simulink model "simulation_Hippocampus_compare_paper"  (R2022b)
settings: Solver=ode3  StartTime=0  StopTime=120  FixedStep=0.001  MaxStep=0.001  MinStep=0.00001  RelTol=1e-5  AbsTol=1e-5  EnableMultiTasking=on
values from neighbouring files (symbols this model uses):
  k_pos_ndi = 8    [parameters.m]
  k_vel_ndi = 8    [parameters.m]
  Kf = 6    [parameters.m]
  Kp = 0.01    [parameters.m]
  Kp_p = 30    [parameters.m]
  Kp_pitch = 8    [parameters.m]
  Kp_q = 10    [parameters.m]
  Kp_r = 10    [parameters.m]
  Kp_roll = 10    [parameters.m]
  Kp_u = 8    [parameters.m]
  Kp_yaw = 8    [parameters.m]
  Kq = 5    [parameters.m]
  Kr = 8    [parameters.m]
  Ktau1 = 0.1    [parameters.m]
  Ktau2 = 5    [parameters.m]
  Ktau3 = 5    [parameters.m]
  Ku = 8    [parameters.m]
  p11 = 0.4    [parameters.m]
  p12 = 0.2    [parameters.m]
  p21 = 0.2    [parameters.m]
  p22 = 0.05    [parameters.m]
  p31 = 0.3    [parameters.m]
  p32 = 0.05    [parameters.m]
  p41 = 0.5    [parameters.m]
  p42 = 0.1    [parameters.m]
  p51 = 0.5    [parameters.m]
  p52 = 0.1    [parameters.m]
  p61 = 0.5    [parameters.m]
  p62 = 0.1    [parameters.m]
  r1 = 4    [parameters.m]
  r2 = 8    [parameters.m]
libraries: simulink x8
(part 1 of 6)
settings Model: Creator=ch  LastModifiedBy=sf
settings SolverCC: MaxConsecutiveZCs=100000  ZeroCrossAlgorithm=Adaptive  AlgebraicLoopSolver=TrustRegion
settings DebuggingCC: MaskedZcDiagnostic=none  IgnoredZcDiagnostic=none  UnconnectedInputMsg=warning  UnconnectedOutputMsg=warning  UnconnectedLineMsg=warning  SFMachineParentedDataDiag=warning  ArithmeticOperatorsInVariantConditions=warning
settings ModelReferenceCC: EnableRefExpFcnMdlSchedulingChecks=on
settings SFSimCC: CustomCodeUndefinedFunction=UseInterfaceOnly
settings RTWCC: DLArmComputeVersion=19.05

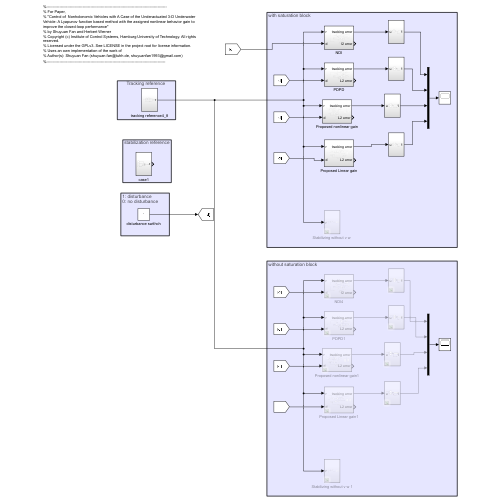
[thumbnail: Simulink's stored preview of the top-level diagram]
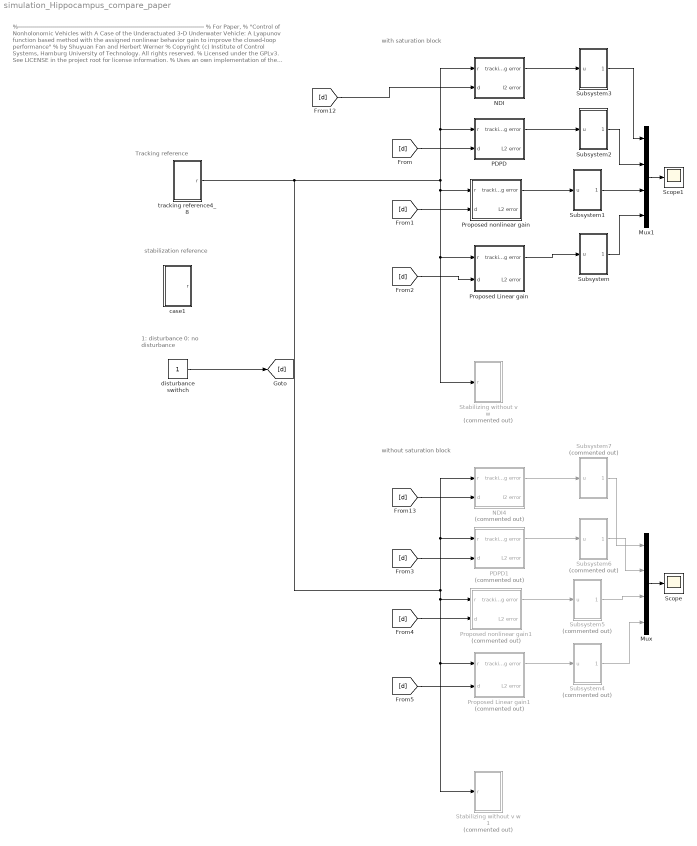
== system simulation_Hippocampus_compare_paper ==
  note: %---------------------------------------------------------------------------------------------
      | % For Paper,
      | % "Control of Nonholonomic Vehicles with A Case of the Underactuated 3-D Underwater Vehicle: A Lyapunov function based method with the assigned nonlinear behavior gain to improve the closed-loop performance"
      | % by Shuyuan Fan and Herbert Werner
      | % Copyright (c) Institute of Control Systems, Hamburg University of Technology. All rights reserved.
      | % Licensed under the GPLv3. See LICENSE in the project root for license information.
      | % Uses an own implementation of the work of
      | % Author(s): Shuyuan Fan (shuyuan.fan@tuhh.de, shuyuanfan1993@gmail.com)
      | %--------------------------------------------------------------------------------------------
  note: Tracking reference
  note: stabilization reference
  note: 1: disturbance
      | 0: no disturbance
  note: with saturation block
  note: without saturation block
  Mux : Mux
  Mux1 : Mux
  NDI : Subsystem
  NDI4 : Subsystem  Commented=on
  PDPD : Subsystem
  PDPD1 : Subsystem  Commented=on
  Proposed Linear gain : Subsystem
  Proposed Linear gain1 : Subsystem  Commented=on
  Proposed nonlinear gain : Subsystem
  Proposed nonlinear gain1 : Subsystem  Commented=on
  Scope : Scope
  Scope1 : Scope
  "Stabilizing without v w " : Subsystem  Commented=on
  Stabilizing without v w 1 : Subsystem  Commented=on
  Subsystem : Subsystem
  Subsystem1 : Subsystem
  Subsystem2 : Subsystem
  Subsystem3 : Subsystem
  Subsystem4 : Subsystem  Commented=on
  Subsystem5 : Subsystem  Commented=on
  Subsystem6 : Subsystem  Commented=on
  Subsystem7 : Subsystem  Commented=on
  case1 : Subsystem
  disturbance swithch : Constant
  tracking reference4_8 : Subsystem
  wires:
  PDPD/1(tracking error) -> Subsystem2/1(u)
  Proposed nonlinear gain/1(tracking error) -> Subsystem1/1(u)
  disturbance swithch/1 -> [d]
  [d] -> PDPD/2(d)
  [d] -> Proposed nonlinear gain/2(d)
  [d] -> Proposed Linear gain/2(d)
  Proposed Linear gain/1(tracking error) -> Subsystem/1(u)
  NDI/1(tracking error) -> Subsystem3/1(u)
  [d] -> Proposed nonlinear gain1/2(d)
  [d] -> Proposed Linear gain1/2(d)
  Proposed Linear gain1/1(tracking error) -> Subsystem4/1(u)
  [d] -> PDPD1/2(d)
  tracking reference4_8/1(r) -> PDPD/1(r), NDI/1(r), "Stabilizing without v w "/1(r), Proposed Linear gain/1(r), Proposed nonlinear gain/1(r), NDI4/1(r), PDPD1/1(r), Stabilizing without v w 1/1(r), Proposed Linear gain1/1(r), Proposed nonlinear gain1/1(r)
  NDI4/1(tracking error) -> Subsystem7/1(u)
  PDPD1/1(tracking error) -> Subsystem6/1(u)
  Proposed nonlinear gain1/1(tracking error) -> Subsystem5/1(u)
  Subsystem6/1(Out1) -> Mux/2
  Subsystem5/1(Out1) -> Mux/3
  Subsystem4/1(Out1) -> Mux/4
  Mux/1 -> Scope/1
  Subsystem2/1(Out1) -> Mux1/2
  Subsystem1/1(Out1) -> Mux1/3
  Subsystem/1(Out1) -> Mux1/4
  Mux1/1 -> Scope1/1
  Subsystem3/1(Out1) -> Mux1/1
  [d] -> NDI/2(d)
  [d] -> NDI4/2(d)
  Subsystem7/1(Out1) -> Mux/1

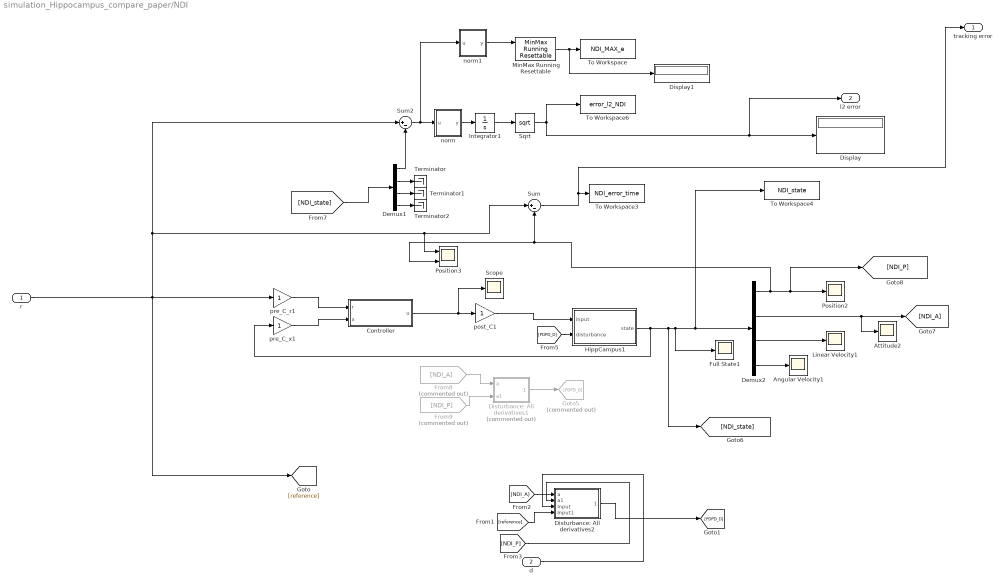
== system simulation_Hippocampus_compare_paper/NDI ==
  r : Inport
  d : Inport  Port=2
  Angular Velocity1 : Scope
  Attitude2 : Scope
  Controller : Subsystem
  Demux1 : Demux  Outputs=[3 3 3 3]
  Demux2 : Demux  Outputs=[3 3 3 3]
  Display : Display
  Display1 : Display
  Disturbance: All derivatives1 : Subsystem  Commented=on
  Disturbance: All derivatives2 : Subsystem
  From8 : From  Commented=on  GotoTag=NDI_A
  From9 : From  Commented=on  GotoTag=NDI_P
  Full State1 : Scope
  Goto5 : Goto  Commented=on  GotoTag=PDPD_D
  HippCampus1 : Subsystem
  Integrator1 : Integrator
  Linear Velocity1 : Scope
  MinMax Running Resettable : simulink/Math Operations/MinMax Running Resettable  Function=max  vinit=0.0
  Position2 : Scope
  Position3 : Scope  NumInputPorts=2
  Scope : Scope
  Sqrt : Sqrt
  Sum : Sum  Inputs=|+-
  Sum2 : Sum  Inputs=|+-
  Terminator : Terminator
  Terminator1 : Terminator
  Terminator2 : Terminator
  To Workspace : ToWorkspace  VariableName=NDI_MAX_e  SaveFormat=Timeseries  SampleTime=-1
  To Workspace3 : ToWorkspace  VariableName=NDI_error_time  SaveFormat=Timeseries  SampleTime=-1
  To Workspace4 : ToWorkspace  VariableName=NDI_state  SaveFormat=Timeseries  SampleTime=-1
  To Workspace6 : ToWorkspace  VariableName=error_l2_NDI  SaveFormat=Timeseries  SampleTime=-1
      settings: MaxDataPoints=1
  norm : MATLAB Function  TreatAsAtomicUnit=on
  norm1 : MATLAB Function  TreatAsAtomicUnit=on
  post_C1 : Gain
  pre_C_r1 : Gain
  pre_C_x1 : Gain
  tracking error : Outport
  l2 error : Outport  Port=2
  wires:
  Controller/1(u) -> post_C1/1, Scope/1
  [PDPD_D] -> HippCampus1/2(disturbance)
  Demux2/2 -> Attitude2/1, [NDI_A]
  HippCampus1/1(state) -> To Workspace4/1, Demux2/1, Full State1/1, [NDI_state], pre_C_x1/1
  pre_C_r1/1 -> Controller/1(r)
  Demux2/3 -> Linear Velocity1/1
  post_C1/1 -> HippCampus1/1(input)
  Disturbance: All derivatives1/1(disturbance) -> Goto5/1
  From9/1 -> Disturbance: All derivatives1/2(a1)
  pre_C_x1/1 -> Controller/2(x)
  Demux2/4 -> Angular Velocity1/1
  From8/1 -> Disturbance: All derivatives1/1(a)
  [NDI_state] -> Demux1/1
  Demux1/3 -> Terminator1/1
  Integrator1/1 -> Sqrt/1
  norm/1(y) -> Integrator1/1
  Demux1/2 -> Terminator/1
  Demux1/1 -> Sum2/2
  Demux1/4 -> Terminator2/1
  Sqrt/1 -> To Workspace6/1, l2 error/1, Display/1
  Sum2/1 -> norm1/1(u), norm/1(u)
  norm1/1(y) -> MinMax Running Resettable/1
  MinMax Running Resettable/1 -> Display1/1, To Workspace/1
  Sum/1 -> tracking error/1, To Workspace3/1
  r/1 -> [reference], Sum/1, Position3/1, Sum2/1, pre_C_r1/1
  Demux2/1 -> [NDI_P], Position2/1, Sum/2, Position3/2
  d/1 -> Disturbance: All derivatives2/3(Input)
  [NDI_P] -> Disturbance: All derivatives2/2(a1)
  [NDI_A] -> Disturbance: All derivatives2/1(a)
  [reference] -> Disturbance: All derivatives2/4(Input1)
  Disturbance: All derivatives2/1(disturbance) -> [PDPD_D]

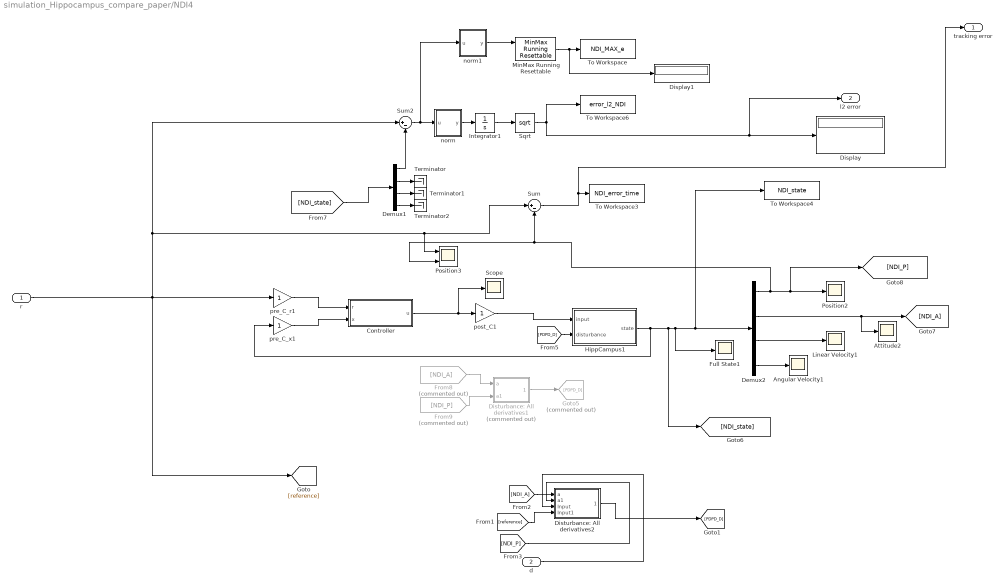
== system simulation_Hippocampus_compare_paper/NDI4 ==
  r : Inport
  d : Inport  Port=2
  Angular Velocity1 : Scope
  Attitude2 : Scope
  Controller : Subsystem
  Demux1 : Demux  Outputs=[3 3 3 3]
  Demux2 : Demux  Outputs=[3 3 3 3]
  Display : Display
  Display1 : Display
  Disturbance: All derivatives1 : Subsystem  Commented=on
  Disturbance: All derivatives2 : Subsystem
  From8 : From  Commented=on  GotoTag=NDI_A
  From9 : From  Commented=on  GotoTag=NDI_P
  Full State1 : Scope
  Goto5 : Goto  Commented=on  GotoTag=PDPD_D
  HippCampus1 : Subsystem
  Integrator1 : Integrator
  Linear Velocity1 : Scope
  MinMax Running Resettable : simulink/Math Operations/MinMax Running Resettable  Function=max  vinit=0.0
  Position2 : Scope
  Position3 : Scope  NumInputPorts=2
  Scope : Scope
  Sqrt : Sqrt
  Sum : Sum  Inputs=|+-
  Sum2 : Sum  Inputs=|+-
  Terminator : Terminator
  Terminator1 : Terminator
  Terminator2 : Terminator
  To Workspace : ToWorkspace  VariableName=NDI_MAX_e  SaveFormat=Timeseries  SampleTime=-1
  To Workspace3 : ToWorkspace  VariableName=NDI_error_time  SaveFormat=Timeseries  SampleTime=-1
  To Workspace4 : ToWorkspace  VariableName=NDI_state  SaveFormat=Timeseries  SampleTime=-1
  To Workspace6 : ToWorkspace  VariableName=error_l2_NDI  SaveFormat=Timeseries  SampleTime=-1
      settings: MaxDataPoints=1
  norm : MATLAB Function  TreatAsAtomicUnit=on
  norm1 : MATLAB Function  TreatAsAtomicUnit=on
  post_C1 : Gain
  pre_C_r1 : Gain
  pre_C_x1 : Gain
  tracking error : Outport
  l2 error : Outport  Port=2
  wires:
  Controller/1(u) -> post_C1/1, Scope/1
  [PDPD_D] -> HippCampus1/2(disturbance)
  Demux2/2 -> Attitude2/1, [NDI_A]
  HippCampus1/1(state) -> To Workspace4/1, Demux2/1, Full State1/1, [NDI_state], pre_C_x1/1
  pre_C_r1/1 -> Controller/1(r)
  Demux2/3 -> Linear Velocity1/1
  post_C1/1 -> HippCampus1/1(input)
  Disturbance: All derivatives1/1(disturbance) -> Goto5/1
  From9/1 -> Disturbance: All derivatives1/2(a1)
  pre_C_x1/1 -> Controller/2(x)
  Demux2/4 -> Angular Velocity1/1
  From8/1 -> Disturbance: All derivatives1/1(a)
  [NDI_state] -> Demux1/1
  Demux1/3 -> Terminator1/1
  Integrator1/1 -> Sqrt/1
  norm/1(y) -> Integrator1/1
  Demux1/2 -> Terminator/1
  Demux1/1 -> Sum2/2
  Demux1/4 -> Terminator2/1
  Sqrt/1 -> To Workspace6/1, l2 error/1, Display/1
  Sum2/1 -> norm1/1(u), norm/1(u)
  norm1/1(y) -> MinMax Running Resettable/1
  MinMax Running Resettable/1 -> Display1/1, To Workspace/1
  Sum/1 -> tracking error/1, To Workspace3/1
  r/1 -> [reference], Sum/1, Position3/1, Sum2/1, pre_C_r1/1
  Demux2/1 -> [NDI_P], Position2/1, Sum/2, Position3/2
  d/1 -> Disturbance: All derivatives2/3(Input)
  [NDI_P] -> Disturbance: All derivatives2/2(a1)
  [NDI_A] -> Disturbance: All derivatives2/1(a)
  [reference] -> Disturbance: All derivatives2/4(Input1)
  Disturbance: All derivatives2/1(disturbance) -> [PDPD_D]

== system simulation_Hippocampus_compare_paper/PDPD ==
  r : Inport
  d : Inport  Port=2
  Angular Velocity1 : Scope
  Attitude2 : Scope
  Controller : Subsystem
  Demux1 : Demux  Outputs=[3 3 3 3]
  Demux2 : Demux  Outputs=[3 3 3 3]
  Display : Display
  Display1 : Display
  Disturbance: All derivatives1 : Subsystem
  Full State1 : Scope
  HippCampus1 : Subsystem
  Integrator1 : Integrator
  Linear Velocity1 : Scope
  MinMax Running Resettable : simulink/Math Operations/MinMax Running Resettable  Function=max  vinit=0.0
  Position2 : Scope
  Position3 : Scope  NumInputPorts=2
  Scope : Scope
  Sqrt : Sqrt
  Sum : Sum  Inputs=|+-
  Sum2 : Sum  Inputs=|+-
  Terminator : Terminator
  Terminator1 : Terminator
  Terminator2 : Terminator
  To Workspace : ToWorkspace  VariableName=PDPD_MAX_e  SaveFormat=Timeseries  SampleTime=-1
  To Workspace1 : ToWorkspace  VariableName=PDPD_error_time  SaveFormat=Timeseries  SampleTime=-1
  To Workspace3 : ToWorkspace  VariableName=PDPD_state  SaveFormat=Timeseries  SampleTime=-1
  To Workspace5 : ToWorkspace  VariableName=error_l2_PDPD  SaveFormat=Timeseries  SampleTime=-1
      settings: MaxDataPoints=1
  norm : MATLAB Function  TreatAsAtomicUnit=on
  norm1 : MATLAB Function  TreatAsAtomicUnit=on
  post_C1 : Gain
  pre_C_r1 : Gain
  pre_C_x1 : Gain
  tracking error : Outport
  L2 error : Outport  Port=2
  wires:
  [PDPD_D] -> HippCampus1/2(disturbance)
  Demux2/2 -> Attitude2/1, [PDPD_A]
  HippCampus1/1(state) -> Full State1/1, Demux2/1, [PDPD_state], To Workspace3/1, pre_C_x1/1
  pre_C_r1/1 -> Controller/1(r)
  Demux2/3 -> Linear Velocity1/1
  post_C1/1 -> Scope/1, HippCampus1/1(input)
  Disturbance: All derivatives1/1(disturbance) -> [PDPD_D]
  [PDPD_P] -> Disturbance: All derivatives1/2(a1)
  pre_C_x1/1 -> Controller/2(x)
  Demux2/4 -> Angular Velocity1/1
  [PDPD_A] -> Disturbance: All derivatives1/1(a)
  [PDPD_state] -> Demux1/1
  Demux1/3 -> Terminator1/1
  Integrator1/1 -> Sqrt/1
  norm/1(y) -> Integrator1/1
  Demux1/2 -> Terminator/1
  Demux1/1 -> Sum2/2
  Demux1/4 -> Terminator2/1
  Sqrt/1 -> L2 error/1, To Workspace5/1, Display/1
  Controller/1(u) -> post_C1/1
  norm1/1(y) -> MinMax Running Resettable/1
  MinMax Running Resettable/1 -> Display1/1, To Workspace/1
  Sum2/1 -> norm1/1(u), norm/1(u)
  Sum/1 -> tracking error/1, To Workspace1/1
  r/1 -> Sum/1, Position3/1, Sum2/1, pre_C_r1/1
  Demux2/1 -> [PDPD_P], Position2/1, Sum/2, Position3/2
  d/1 -> Disturbance: All derivatives1/3(Input)

== system simulation_Hippocampus_compare_paper/PDPD1 ==
  r : Inport
  d : Inport  Port=2
  Angular Velocity1 : Scope
  Attitude2 : Scope
  Controller : Subsystem
  Demux1 : Demux  Outputs=[3 3 3 3]
  Demux2 : Demux  Outputs=[3 3 3 3]
  Display : Display
  Display1 : Display
  Disturbance: All derivatives1 : Subsystem
  Full State1 : Scope
  HippCampus1 : Subsystem
  Integrator1 : Integrator
  Linear Velocity1 : Scope
  MinMax Running Resettable : simulink/Math Operations/MinMax Running Resettable  Function=max  vinit=0.0
  Position2 : Scope
  Position3 : Scope  NumInputPorts=2
  Scope : Scope
  Sqrt : Sqrt
  Sum : Sum  Inputs=|+-
  Sum2 : Sum  Inputs=|+-
  Terminator : Terminator
  Terminator1 : Terminator
  Terminator2 : Terminator
  To Workspace : ToWorkspace  VariableName=PDPD_MAX_e  SaveFormat=Timeseries  SampleTime=-1
  To Workspace1 : ToWorkspace  VariableName=PDPD_error_time  SaveFormat=Timeseries  SampleTime=-1
  To Workspace3 : ToWorkspace  VariableName=PDPD_state  SaveFormat=Timeseries  SampleTime=-1
  To Workspace5 : ToWorkspace  VariableName=error_l2_PDPD  SaveFormat=Timeseries  SampleTime=-1
      settings: MaxDataPoints=1
  norm : MATLAB Function  TreatAsAtomicUnit=on
  norm1 : MATLAB Function  TreatAsAtomicUnit=on
  post_C1 : Gain
  pre_C_r1 : Gain
  pre_C_x1 : Gain
  tracking error : Outport
  L2 error : Outport  Port=2
  wires:
  [PDPD_D] -> HippCampus1/2(disturbance)
  Demux2/2 -> Attitude2/1, [PDPD_A]
  HippCampus1/1(state) -> Full State1/1, Demux2/1, [PDPD_state], To Workspace3/1, pre_C_x1/1
  pre_C_r1/1 -> Controller/1(r)
  Demux2/3 -> Linear Velocity1/1
  post_C1/1 -> Scope/1, HippCampus1/1(input)
  Disturbance: All derivatives1/1(disturbance) -> [PDPD_D]
  [PDPD_P] -> Disturbance: All derivatives1/2(a1)
  pre_C_x1/1 -> Controller/2(x)
  Demux2/4 -> Angular Velocity1/1
  [PDPD_A] -> Disturbance: All derivatives1/1(a)
  [PDPD_state] -> Demux1/1
  Demux1/3 -> Terminator1/1
  Integrator1/1 -> Sqrt/1
  norm/1(y) -> Integrator1/1
  Demux1/2 -> Terminator/1
  Demux1/1 -> Sum2/2
  Demux1/4 -> Terminator2/1
  Sqrt/1 -> L2 error/1, To Workspace5/1, Display/1
  Controller/1(u) -> post_C1/1
  norm1/1(y) -> MinMax Running Resettable/1
  MinMax Running Resettable/1 -> Display1/1, To Workspace/1
  Sum2/1 -> norm1/1(u), norm/1(u)
  Sum/1 -> tracking error/1, To Workspace1/1
  r/1 -> Sum/1, Position3/1, Sum2/1, pre_C_r1/1
  Demux2/1 -> [PDPD_P], Position2/1, Sum/2, Position3/2
  d/1 -> Disturbance: All derivatives1/3(Input)

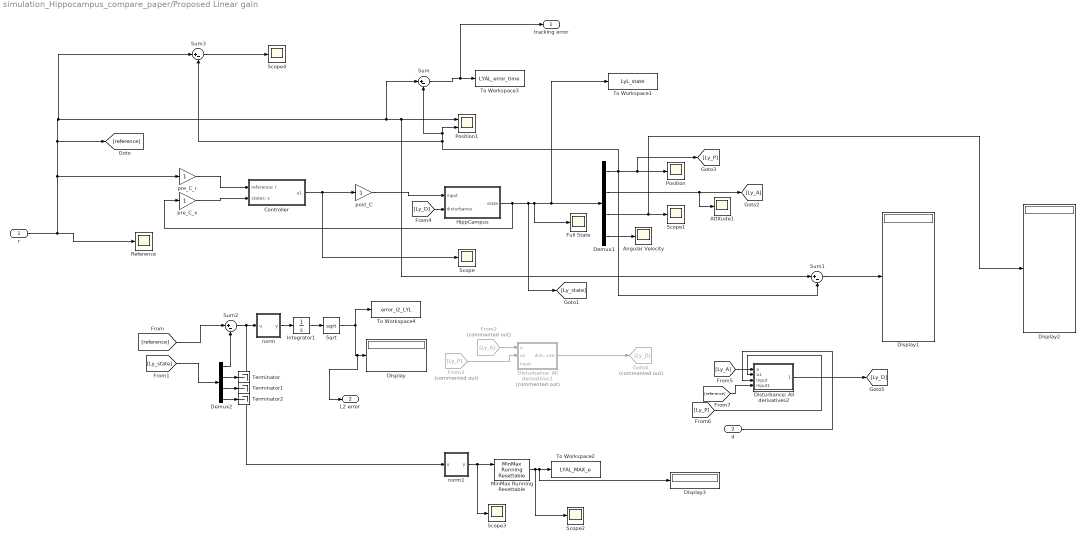
== system simulation_Hippocampus_compare_paper/Proposed Linear gain ==
  r : Inport
  d : Inport  Port=2
  Angular Velocity : Scope
  Attitude1 : Scope
  Controller : Subsystem
  Demux1 : Demux  Outputs=[3 3 3 3]
  Demux2 : Demux  Outputs=[3 3 3 3]
  Display{,1..3} (4 alike) : Display
  Disturbance: All derivatives1 : Subsystem  Commented=on
  Disturbance: All derivatives2 : Subsystem
  From2 : From  Commented=on  GotoTag=Ly_A
  From3 : From  Commented=on  GotoTag=Ly_P
  Full State : Scope
  Goto4 : Goto  Commented=on  GotoTag=Ly_D
  HippCampus : Subsystem
  Integrator1 : Integrator
  MinMax Running Resettable : simulink/Math Operations/MinMax Running Resettable  Function=max  vinit=0.0
  Position : Scope
  Position1 : Scope  NumInputPorts=2
  Reference : Scope
  Scope{,1..4} (5 alike) : Scope
  Sqrt : Sqrt
  Sum{,1..3} (4 alike) : Sum  Inputs=|+-
  Terminator : Terminator
  Terminator1 : Terminator
  Terminator2 : Terminator
  To Workspace1 : ToWorkspace  VariableName=LyL_state  SaveFormat=Timeseries  SampleTime=-1
  To Workspace2 : ToWorkspace  VariableName=LYAL_MAX_e  SaveFormat=Timeseries  SampleTime=-1
  To Workspace3 : ToWorkspace  VariableName=LYAL_error_time  SaveFormat=Timeseries  SampleTime=-1
  To Workspace4 : ToWorkspace  VariableName=error_l2_LYL  SaveFormat=Timeseries  SampleTime=-1
      settings: MaxDataPoints=1
  norm : MATLAB Function  TreatAsAtomicUnit=on
  norm1 : MATLAB Function  TreatAsAtomicUnit=on
  post_C : Gain
  pre_C_r : Gain
  pre_C_x : Gain
  tracking error : Outport
  L2 error : Outport  Port=2
  wires:
  HippCampus/1(state) -> To Workspace1/1, Demux1/1, Full State/1, [Ly_state], pre_C_x/1
  Disturbance: All derivatives1/1(disturbance) -> Goto4/1
  Demux1/3 -> Scope1/1, Display2/1
  Demux2/3 -> Terminator1/1
  [Ly_state] -> Demux2/1
  Controller/1(u1) -> Scope/1, post_C/1
  [reference] -> Sum2/1
  Demux2/1 -> Sum2/2
  norm/1(y) -> Integrator1/1
  pre_C_x/1 -> Controller/2(states: x)
  Integrator1/1 -> Sqrt/1
  Sqrt/1 -> To Workspace4/1, L2 error/1, Display/1
  Demux1/4 -> Angular Velocity/1
  [Ly_D] -> HippCampus/2(disturbance)
  Demux1/2 -> Attitude1/1, [Ly_A]
  pre_C_r/1 -> Controller/1(reference: r)
  Demux2/4 -> Terminator2/1
  Demux1/1 -> [Ly_P], Position/1, Sum3/2, Sum/2, Position1/2, Sum1/2
  post_C/1 -> HippCampus/1(input)
  From3/1 -> Disturbance: All derivatives1/2(a1)
  Demux2/2 -> Terminator/1
  From2/1 -> Disturbance: All derivatives1/1(a)
  Sum2/1 -> norm/1(u), norm1/1(u)
  MinMax Running Resettable/1 -> Scope2/1, Display3/1, To Workspace2/1
  norm1/1(y) -> Scope3/1, MinMax Running Resettable/1
  Sum/1 -> tracking error/1, To Workspace3/1
  r/1 -> Sum3/1, Sum/1, Sum1/1, Position1/1, [reference], pre_C_r/1, Reference/1
  Sum1/1 -> Display1/1
  Sum3/1 -> Scope4/1
  ? -> Disturbance: All derivatives1/3(Input)
  [reference] -> Disturbance: All derivatives2/4(Input1)
  d/1 -> Disturbance: All derivatives2/3(Input)
  [Ly_A] -> Disturbance: All derivatives2/1(a)
  [Ly_P] -> Disturbance: All derivatives2/2(a1)
  Disturbance: All derivatives2/1(disturbance) -> [Ly_D]

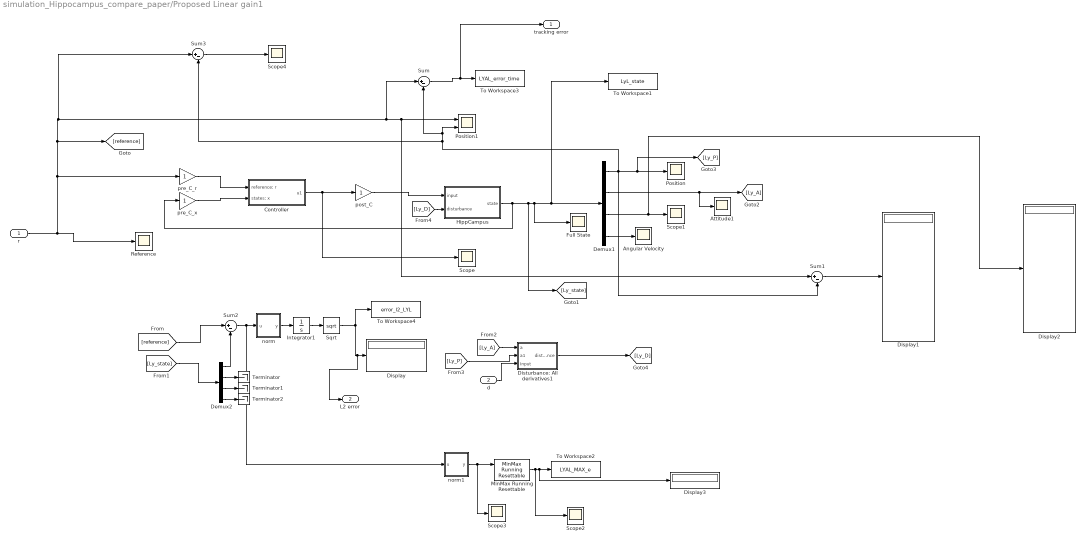
== system simulation_Hippocampus_compare_paper/Proposed Linear gain1 ==
  r : Inport
  d : Inport  Port=2
  Angular Velocity : Scope
  Attitude1 : Scope
  Controller : Subsystem
  Demux1 : Demux  Outputs=[3 3 3 3]
  Demux2 : Demux  Outputs=[3 3 3 3]
  Display{,1..3} (4 alike) : Display
  Disturbance: All derivatives1 : Subsystem
  Full State : Scope
  HippCampus : Subsystem
  Integrator1 : Integrator
  MinMax Running Resettable : simulink/Math Operations/MinMax Running Resettable  Function=max  vinit=0.0
  Position : Scope
  Position1 : Scope  NumInputPorts=2
  Reference : Scope
  Scope{,1..4} (5 alike) : Scope
  Sqrt : Sqrt
  Sum{,1..3} (4 alike) : Sum  Inputs=|+-
  Terminator : Terminator
  Terminator1 : Terminator
  Terminator2 : Terminator
  To Workspace1 : ToWorkspace  VariableName=LyL_state  SaveFormat=Timeseries  SampleTime=-1
  To Workspace2 : ToWorkspace  VariableName=LYAL_MAX_e  SaveFormat=Timeseries  SampleTime=-1
  To Workspace3 : ToWorkspace  VariableName=LYAL_error_time  SaveFormat=Timeseries  SampleTime=-1
  To Workspace4 : ToWorkspace  VariableName=error_l2_LYL  SaveFormat=Timeseries  SampleTime=-1
      settings: MaxDataPoints=1
  norm : MATLAB Function  TreatAsAtomicUnit=on
  norm1 : MATLAB Function  TreatAsAtomicUnit=on
  post_C : Gain
  pre_C_r : Gain
  pre_C_x : Gain
  tracking error : Outport
  L2 error : Outport  Port=2
  wires:
  HippCampus/1(state) -> To Workspace1/1, Demux1/1, Full State/1, [Ly_state], pre_C_x/1
  Disturbance: All derivatives1/1(disturbance) -> [Ly_D]
  Demux1/3 -> Scope1/1, Display2/1
  Demux2/3 -> Terminator1/1
  [Ly_state] -> Demux2/1
  Controller/1(u1) -> Scope/1, post_C/1
  [reference] -> Sum2/1
  Demux2/1 -> Sum2/2
  norm/1(y) -> Integrator1/1
  pre_C_x/1 -> Controller/2(states: x)
  Integrator1/1 -> Sqrt/1
  Sqrt/1 -> To Workspace4/1, L2 error/1, Display/1
  Demux1/4 -> Angular Velocity/1
  [Ly_D] -> HippCampus/2(disturbance)
  Demux1/2 -> Attitude1/1, [Ly_A]
  pre_C_r/1 -> Controller/1(reference: r)
  Demux2/4 -> Terminator2/1
  Demux1/1 -> [Ly_P], Position/1, Sum3/2, Sum/2, Position1/2, Sum1/2
  post_C/1 -> HippCampus/1(input)
  [Ly_P] -> Disturbance: All derivatives1/2(a1)
  Demux2/2 -> Terminator/1
  [Ly_A] -> Disturbance: All derivatives1/1(a)
  Sum2/1 -> norm/1(u), norm1/1(u)
  MinMax Running Resettable/1 -> Scope2/1, Display3/1, To Workspace2/1
  norm1/1(y) -> Scope3/1, MinMax Running Resettable/1
  Sum/1 -> tracking error/1, To Workspace3/1
  r/1 -> Sum3/1, Sum/1, Sum1/1, Position1/1, [reference], pre_C_r/1, Reference/1
  Sum1/1 -> Display1/1
  Sum3/1 -> Scope4/1
  d/1 -> Disturbance: All derivatives1/3(Input)

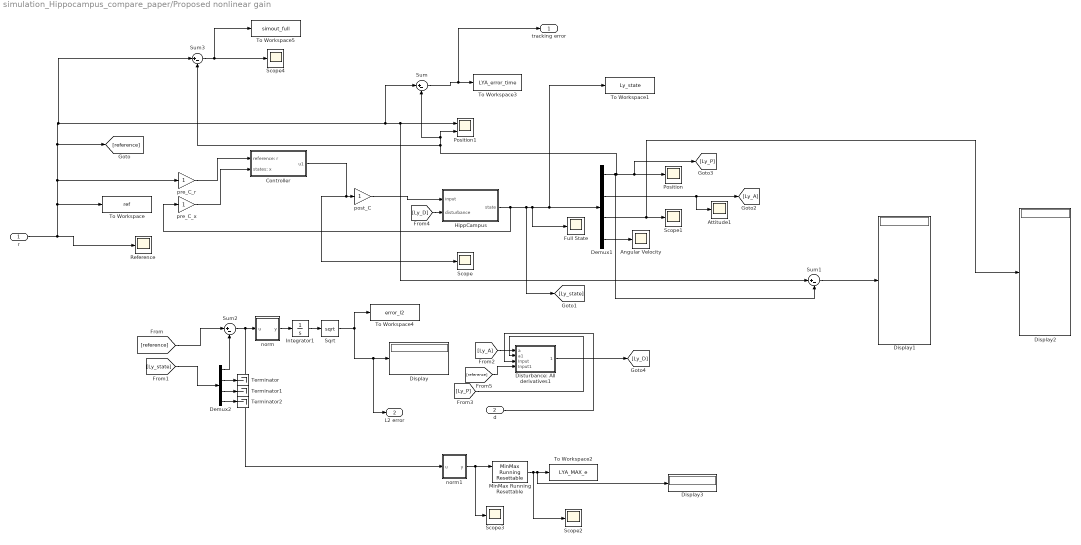
== system simulation_Hippocampus_compare_paper/Proposed nonlinear gain ==
  r : Inport
  d : Inport  Port=2
  Angular Velocity : Scope
  Attitude1 : Scope
  Controller : Subsystem
  Demux1 : Demux  Outputs=[3 3 3 3]
  Demux2 : Demux  Outputs=[3 3 3 3]
  Display{,1..3} (4 alike) : Display
  Disturbance: All derivatives1 : Subsystem
  Full State : Scope
  HippCampus : Subsystem
  Integrator1 : Integrator
  MinMax Running Resettable : simulink/Math Operations/MinMax Running Resettable  Function=max  vinit=0.0
  Position : Scope
  Position1 : Scope  NumInputPorts=2
  Reference : Scope
  Scope{,1..4} (5 alike) : Scope
  Sqrt : Sqrt
  Sum{,1..3} (4 alike) : Sum  Inputs=|+-
  Terminator : Terminator
  Terminator1 : Terminator
  Terminator2 : Terminator
  To Workspace : ToWorkspace  VariableName=ref  SaveFormat=Timeseries  SampleTime=-1
  To Workspace1 : ToWorkspace  VariableName=Ly_state  SaveFormat=Timeseries  SampleTime=-1
  To Workspace2 : ToWorkspace  VariableName=LYA_MAX_e  SaveFormat=Timeseries  SampleTime=-1
  To Workspace3 : ToWorkspace  VariableName=LYA_error_time  SaveFormat=Timeseries  SampleTime=-1
  To Workspace4 : ToWorkspace  VariableName=error_l2  SaveFormat=Timeseries  SampleTime=-1
      settings: MaxDataPoints=1
  To Workspace5 : ToWorkspace  VariableName=simout_full  SaveFormat=Timeseries  SampleTime=-1
  norm : MATLAB Function  TreatAsAtomicUnit=on
  norm1 : MATLAB Function  TreatAsAtomicUnit=on
  post_C : Gain
  pre_C_r : Gain
  pre_C_x : Gain
  tracking error : Outport
  L2 error : Outport  Port=2
  wires:
  HippCampus/1(state) -> To Workspace1/1, Demux1/1, Full State/1, [Ly_state], pre_C_x/1
  Disturbance: All derivatives1/1(disturbance) -> [Ly_D]
  Demux1/3 -> Scope1/1, Display2/1
  Demux2/3 -> Terminator1/1
  [Ly_state] -> Demux2/1
  Controller/1(u1) -> Scope/1, post_C/1
  [reference] -> Sum2/1
  Demux2/1 -> Sum2/2
  norm/1(y) -> Integrator1/1
  pre_C_x/1 -> Controller/2(states: x)
  Integrator1/1 -> Sqrt/1
  Sqrt/1 -> To Workspace4/1, L2 error/1, Display/1
  Demux1/4 -> Angular Velocity/1
  [Ly_D] -> HippCampus/2(disturbance)
  Demux1/2 -> Attitude1/1, [Ly_A]
  pre_C_r/1 -> Controller/1(reference: r)
  Demux2/4 -> Terminator2/1
  Demux1/1 -> [Ly_P], Position/1, Sum3/2, Sum/2, Position1/2, Sum1/2
  post_C/1 -> HippCampus/1(input)
  [Ly_P] -> Disturbance: All derivatives1/2(a1)
  Demux2/2 -> Terminator/1
  [Ly_A] -> Disturbance: All derivatives1/1(a)
  Sum2/1 -> norm/1(u), norm1/1(u)
  MinMax Running Resettable/1 -> Scope2/1, Display3/1, To Workspace2/1
  norm1/1(y) -> Scope3/1, MinMax Running Resettable/1
  Sum/1 -> tracking error/1, To Workspace3/1
  r/1 -> Sum3/1, Sum/1, Sum1/1, Position1/1, [reference], pre_C_r/1, To Workspace/1, Reference/1
  Sum1/1 -> Display1/1
  Sum3/1 -> To Workspace5/1, Scope4/1
  d/1 -> Disturbance: All derivatives1/3(Input)
  [reference] -> Disturbance: All derivatives1/4(Input1)

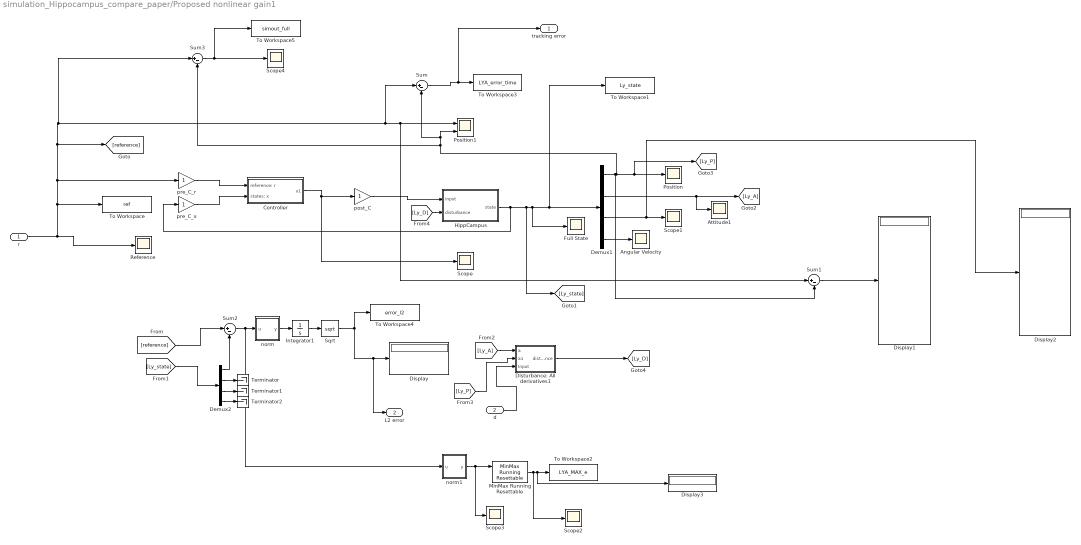
== system simulation_Hippocampus_compare_paper/Proposed nonlinear gain1 ==
  r : Inport
  d : Inport  Port=2
  Angular Velocity : Scope
  Attitude1 : Scope
  Controller : Subsystem
  Demux1 : Demux  Outputs=[3 3 3 3]
  Demux2 : Demux  Outputs=[3 3 3 3]
  Display{,1..3} (4 alike) : Display
  Disturbance: All derivatives1 : Subsystem
  Full State : Scope
  HippCampus : Subsystem
  Integrator1 : Integrator
  MinMax Running Resettable : simulink/Math Operations/MinMax Running Resettable  Function=max  vinit=0.0
  Position : Scope
  Position1 : Scope  NumInputPorts=2
  Reference : Scope
  Scope{,1..4} (5 alike) : Scope
  Sqrt : Sqrt
  Sum{,1..3} (4 alike) : Sum  Inputs=|+-
  Terminator : Terminator
  Terminator1 : Terminator
  Terminator2 : Terminator
  To Workspace : ToWorkspace  VariableName=ref  SaveFormat=Timeseries  SampleTime=-1
  To Workspace1 : ToWorkspace  VariableName=Ly_state  SaveFormat=Timeseries  SampleTime=-1
  To Workspace2 : ToWorkspace  VariableName=LYA_MAX_e  SaveFormat=Timeseries  SampleTime=-1
  To Workspace3 : ToWorkspace  VariableName=LYA_error_time  SaveFormat=Timeseries  SampleTime=-1
  To Workspace4 : ToWorkspace  VariableName=error_l2  SaveFormat=Timeseries  SampleTime=-1
      settings: MaxDataPoints=1
  To Workspace5 : ToWorkspace  VariableName=simout_full  SaveFormat=Timeseries  SampleTime=-1
  norm : MATLAB Function  TreatAsAtomicUnit=on
  norm1 : MATLAB Function  TreatAsAtomicUnit=on
  post_C : Gain
  pre_C_r : Gain
  pre_C_x : Gain
  tracking error : Outport
  L2 error : Outport  Port=2
  wires:
  HippCampus/1(state) -> To Workspace1/1, Demux1/1, Full State/1, [Ly_state], pre_C_x/1
  Disturbance: All derivatives1/1(disturbance) -> [Ly_D]
  Demux1/3 -> Scope1/1, Display2/1
  Demux2/3 -> Terminator1/1
  [Ly_state] -> Demux2/1
  Controller/1(u1) -> Scope/1, post_C/1
  [reference] -> Sum2/1
  Demux2/1 -> Sum2/2
  norm/1(y) -> Integrator1/1
  pre_C_x/1 -> Controller/2(states: x)
  Integrator1/1 -> Sqrt/1
  Sqrt/1 -> To Workspace4/1, L2 error/1, Display/1
  Demux1/4 -> Angular Velocity/1
  [Ly_D] -> HippCampus/2(disturbance)
  Demux1/2 -> Attitude1/1, [Ly_A]
  pre_C_r/1 -> Controller/1(reference: r)
  Demux2/4 -> Terminator2/1
  Demux1/1 -> [Ly_P], Position/1, Sum3/2, Sum/2, Position1/2, Sum1/2
  post_C/1 -> HippCampus/1(input)
  [Ly_P] -> Disturbance: All derivatives1/2(a1)
  Demux2/2 -> Terminator/1
  [Ly_A] -> Disturbance: All derivatives1/1(a)
  Sum2/1 -> norm/1(u), norm1/1(u)
  MinMax Running Resettable/1 -> Scope2/1, Display3/1, To Workspace2/1
  norm1/1(y) -> Scope3/1, MinMax Running Resettable/1
  Sum/1 -> tracking error/1, To Workspace3/1
  r/1 -> Sum3/1, Sum/1, Sum1/1, Position1/1, [reference], pre_C_r/1, To Workspace/1, Reference/1
  Sum1/1 -> Display1/1
  Sum3/1 -> To Workspace5/1, Scope4/1
  d/1 -> Disturbance: All derivatives1/3(Input)

== system simulation_Hippocampus_compare_paper/Stabilizing without v w  ==
  r : Inport
  Angular Velocity : Scope
  Attitude1 : Scope
  Controller : Subsystem
  Demux1 : Demux  Outputs=[3 3 3 3]
  Display1 : Display
  Display2 : Display
  Full State : Scope
  HippCampus : Subsystem
  Position : Scope
  Position1 : Scope  NumInputPorts=2
  Reference : Scope
  Scope : Scope
  Scope1 : Scope
  Scope2 : Scope
  Sum : Sum  Inputs=|+-
  Sum1 : Sum  Inputs=|+-
  To Workspace1 : ToWorkspace  VariableName=simout_novw  SaveFormat=Timeseries  SampleTime=-1
  post_C : Gain
  pre_C_r : Gain
  pre_C_x : Gain
  wires:
  HippCampus/1(state) -> Demux1/1, Full State/1, pre_C_x/1
  Demux1/3 -> Scope1/1, Display2/1
  Controller/1(u1) -> post_C/1, Scope/1
  pre_C_x/1 -> Controller/2(states: x)
  Demux1/4 -> Angular Velocity/1
  [Ly_D] -> HippCampus/2(disturbance)
  Demux1/2 -> Attitude1/1
  pre_C_r/1 -> Controller/1(reference: r)
  Demux1/1 -> Sum/2, Position1/2, Position/1, Sum1/2
  post_C/1 -> HippCampus/1(input)
  r/1 -> Sum/1, Sum1/1, Position1/1, pre_C_r/1, Reference/1
  Sum1/1 -> Display1/1
  Sum/1 -> To Workspace1/1, Scope2/1

== system simulation_Hippocampus_compare_paper/Stabilizing without v w 1 ==
  r : Inport
  Angular Velocity : Scope
  Attitude1 : Scope
  Controller : Subsystem
  Demux1 : Demux  Outputs=[3 3 3 3]
  Display1 : Display
  Display2 : Display
  Full State : Scope
  HippCampus : Subsystem
  Position : Scope
  Position1 : Scope  NumInputPorts=2
  Reference : Scope
  Scope : Scope
  Scope1 : Scope
  Scope2 : Scope
  Sum : Sum  Inputs=|+-
  Sum1 : Sum  Inputs=|+-
  To Workspace1 : ToWorkspace  VariableName=simout_novw  SaveFormat=Timeseries  SampleTime=-1
  post_C : Gain
  pre_C_r : Gain
  pre_C_x : Gain
  wires:
  HippCampus/1(state) -> Demux1/1, Full State/1, pre_C_x/1
  Demux1/3 -> Scope1/1, Display2/1
  Controller/1(u1) -> post_C/1, Scope/1
  pre_C_x/1 -> Controller/2(x)
  Demux1/4 -> Angular Velocity/1
  [Ly_D] -> HippCampus/2(disturbance)
  Demux1/2 -> Attitude1/1
  pre_C_r/1 -> Controller/1(In4)
  Demux1/1 -> Sum/2, Position1/2, Position/1, Sum1/2
  post_C/1 -> HippCampus/1(input)
  r/1 -> Sum/1, Sum1/1, Position1/1, pre_C_r/1, Reference/1
  Sum1/1 -> Display1/1
  Sum/1 -> To Workspace1/1, Scope2/1

== system simulation_Hippocampus_compare_paper/Subsystem ==
  u : Inport
  MATLAB Function3 : MATLAB Function  TreatAsAtomicUnit=on
  MATLAB Function6 : MATLAB Function  TreatAsAtomicUnit=on
  Mux2 : Mux  Inputs=2
  To Workspace : ToWorkspace  VariableName=Proposed_Linear_norm_error  SaveFormat=Timeseries  SampleTime=-1
  Out1 : Outport
  wires:
  MATLAB Function3/1(y) -> Mux2/1
  u/1 -> MATLAB Function6/1(u), MATLAB Function3/1(u)
  MATLAB Function6/1(y) -> Mux2/2
  Mux2/1 -> Out1/1, To Workspace/1

== system simulation_Hippocampus_compare_paper/Subsystem1 ==
  u : Inport
  MATLAB Function3 : MATLAB Function  TreatAsAtomicUnit=on
  MATLAB Function6 : MATLAB Function  TreatAsAtomicUnit=on
  Mux2 : Mux  Inputs=2
  To Workspace : ToWorkspace  VariableName=Proposed_Nonlinear_norm_error  SaveFormat=Timeseries  SampleTime=-1
  Out1 : Outport
  wires:
  MATLAB Function3/1(y) -> Mux2/1
  u/1 -> MATLAB Function6/1(u), MATLAB Function3/1(u)
  MATLAB Function6/1(y) -> Mux2/2
  Mux2/1 -> Out1/1, To Workspace/1

== system simulation_Hippocampus_compare_paper/Subsystem2 ==
  u : Inport
  MATLAB Function3 : MATLAB Function  TreatAsAtomicUnit=on
  MATLAB Function6 : MATLAB Function  TreatAsAtomicUnit=on
  Mux2 : Mux  Inputs=2
  To Workspace : ToWorkspace  VariableName=PDPD_norm_error  SaveFormat=Timeseries  SampleTime=-1
  Out1 : Outport
  wires:
  MATLAB Function3/1(y) -> Mux2/1
  u/1 -> MATLAB Function6/1(u), MATLAB Function3/1(u)
  MATLAB Function6/1(y) -> Mux2/2
  Mux2/1 -> Out1/1, To Workspace/1

== system simulation_Hippocampus_compare_paper/Subsystem3 ==
  u : Inport
  MATLAB Function3 : MATLAB Function  TreatAsAtomicUnit=on
  MATLAB Function6 : MATLAB Function  TreatAsAtomicUnit=on
  Mux2 : Mux  Inputs=2
  To Workspace : ToWorkspace  VariableName=NDI_norm_error  SaveFormat=Timeseries  SampleTime=-1
  Out1 : Outport
  wires:
  MATLAB Function3/1(y) -> Mux2/1
  u/1 -> MATLAB Function6/1(u), MATLAB Function3/1(u)
  MATLAB Function6/1(y) -> Mux2/2
  Mux2/1 -> Out1/1, To Workspace/1

== system simulation_Hippocampus_compare_paper/Subsystem4 ==
  u : Inport
  MATLAB Function3 : MATLAB Function  TreatAsAtomicUnit=on
  MATLAB Function6 : MATLAB Function  TreatAsAtomicUnit=on
  Mux2 : Mux  Inputs=2
  To Workspace : ToWorkspace  VariableName=Proposed_Linear_norm_error  SaveFormat=Timeseries  SampleTime=-1
  Out1 : Outport
  wires:
  MATLAB Function3/1(y) -> Mux2/1
  u/1 -> MATLAB Function6/1(u), MATLAB Function3/1(u)
  MATLAB Function6/1(y) -> Mux2/2
  Mux2/1 -> Out1/1, To Workspace/1

== system simulation_Hippocampus_compare_paper/Subsystem5 ==
  u : Inport
  MATLAB Function3 : MATLAB Function  TreatAsAtomicUnit=on
  MATLAB Function6 : MATLAB Function  TreatAsAtomicUnit=on
  Mux2 : Mux  Inputs=2
  To Workspace : ToWorkspace  VariableName=Proposed_Nonlinear_norm_error  SaveFormat=Timeseries  SampleTime=-1
  Out1 : Outport
  wires:
  MATLAB Function3/1(y) -> Mux2/1
  u/1 -> MATLAB Function6/1(u), MATLAB Function3/1(u)
  MATLAB Function6/1(y) -> Mux2/2
  Mux2/1 -> Out1/1, To Workspace/1

== system simulation_Hippocampus_compare_paper/Subsystem6 ==
  u : Inport
  MATLAB Function3 : MATLAB Function  TreatAsAtomicUnit=on
  MATLAB Function6 : MATLAB Function  TreatAsAtomicUnit=on
  Mux2 : Mux  Inputs=2
  To Workspace : ToWorkspace  VariableName=PDPD_norm_error  SaveFormat=Timeseries  SampleTime=-1
  Out1 : Outport
  wires:
  MATLAB Function3/1(y) -> Mux2/1
  u/1 -> MATLAB Function6/1(u), MATLAB Function3/1(u)
  MATLAB Function6/1(y) -> Mux2/2
  Mux2/1 -> Out1/1, To Workspace/1

== system simulation_Hippocampus_compare_paper/Subsystem7 ==
  u : Inport
  MATLAB Function3 : MATLAB Function  TreatAsAtomicUnit=on
  MATLAB Function6 : MATLAB Function  TreatAsAtomicUnit=on
  Mux2 : Mux  Inputs=2
  To Workspace : ToWorkspace  VariableName=NDI_norm_error  SaveFormat=Timeseries  SampleTime=-1
  Out1 : Outport
  wires:
  MATLAB Function3/1(y) -> Mux2/1
  u/1 -> MATLAB Function6/1(u), MATLAB Function3/1(u)
  MATLAB Function6/1(y) -> Mux2/2
  Mux2/1 -> Out1/1, To Workspace/1

== system simulation_Hippocampus_compare_paper/case1 ==
  Constant : Constant  Value=-1.5
  Constant1 : Constant  Value=-0.8
  Constant2 : Constant  Value=1.2
  Mux3 : Mux  Inputs=[1 1 1]
  r : Outport
  wires:
  Constant1/1 -> Mux3/3
  Constant2/1 -> Mux3/1
  Constant/1 -> Mux3/2
  Mux3/1 -> r/1  "r"

== system simulation_Hippocampus_compare_paper/tracking reference4_8 ==
  Clock : Clock
  Cos : Trigonometry
  Cos1 : Trigonometry
  Gain5 : Gain  Gain=0.1
  Gain6 : Gain  Gain=r1
  Gain7 : Gain  Gain=r2
  Gain8 : Gain  Gain=pi/15
  Gain9 : Gain  Gain=pi/30
  Mux : Mux  Inputs=3
  r : Outport
  wires:
  Gain9/1 -> Cos/1
  Gain6/1 -> Mux/1
  Gain7/1 -> Mux/2
  Cos1/1 -> Gain6/1
  Cos/1 -> Gain7/1
  Mux/1 -> r/1  "r"
  Gain8/1 -> Cos1/1
  Gain5/1 -> Mux/3
  Clock/1 -> Gain5/1, Gain9/1, Gain8/1

== system simulation_Hippocampus_compare_paper/NDI/Controller ==
  r : Inport
  x : Inport  Port=2
  Constant : Constant  Value=k_pos_ndi
  Constant1 : Constant  Value=k_vel_ndi
  Demux1 : Demux  Outputs=[3 3 3 3]
  Gain : Gain  Gain=[ eye(3); zeros(3) ]  Multiplication=Matrix(K*u) (u vector)
  MATLAB Function : MATLAB Function  TreatAsAtomicUnit=on
  Mux1 : Mux  Inputs=2
  Pos controller1 : MATLAB Function  TreatAsAtomicUnit=on
  Saturation : Saturate  UpperLimit=6  LowerLimit=-6
  Scope : Scope
  Subsystem : Subsystem
  Subsystem1 : Subsystem
  Terminator1 : Terminator
  Terminator4 : Terminator
  u : Outport
  wires:
  Subsystem/1(tau) -> u/1
  Constant/1 -> Pos controller1/3(k_pos)
  r/1 -> Gain/1
  Constant1/1 -> Pos controller1/4(k_vel)
  Demux1/3 -> Mux1/2
  Subsystem1/1(x_2pi) -> Demux1/1, MATLAB Function/2(x), Subsystem/3(state)
  Mux1/1 -> Pos controller1/2(x)
  Gain/1 -> Pos controller1/1(r)
  Demux1/1 -> Mux1/1
  Pos controller1/1(u) -> Scope/1, Saturation/1
  Pos controller1/2(theta_des) -> MATLAB Function/1("theta_des ")
  Demux1/2 -> Terminator4/1
  Demux1/4 -> Terminator1/1
  x/1 -> Subsystem1/1(x)
  MATLAB Function/1(theta_des) -> Subsystem/2(rpy_ref)
  Saturation/1 -> Subsystem/1(u_ref)

== system simulation_Hippocampus_compare_paper/NDI/Disturbance: All derivatives1 ==
  a : Inport
  a1 : Inport  Port=2
  Gain1 : Gain  Gain=0  Multiplication=Matrix(K*u)
  Gain2 : Gain  Multiplication=Matrix(K*u)
  Gain3 : Gain  Gain=0  Multiplication=Matrix(K*u)
  Sum2 : Sum  Inputs=|+++
  disturbance2 : Subsystem
  disturbance3 : Subsystem
  old disturbance : Subsystem
  disturbance : Outport
  wires:
  Sum2/1 -> disturbance/1
  Gain1/1 -> Sum2/1
  disturbance2/1(Out1) -> Gain2/1
  a/1 -> disturbance3/1(a)
  a1/1 -> disturbance3/2(a1)
  disturbance3/1(d) -> Gain1/1
  Gain2/1 -> Sum2/2
  old disturbance/1(Out1) -> Gain3/1
  Gain3/1 -> Sum2/3

== system simulation_Hippocampus_compare_paper/NDI/Disturbance: All derivatives2 ==
  a : Inport
  a1 : Inport  Port=2
  Input : Inport  Port=3
  Input1 : Inport  Port=4
  Gain1 : Gain  Gain=0  Multiplication=Matrix(K*u)
  Gain2 : Gain  Multiplication=Matrix(K*u)
  Gain3 : Gain  Gain=0  Multiplication=Matrix(K*u)
  Gain4 : Gain  Gain=0  Multiplication=Matrix(K*u)
  MATLAB Function : MATLAB Function  TreatAsAtomicUnit=on
  MATLAB Function1 : MATLAB Function  TreatAsAtomicUnit=on
  Scope : Scope
  Sum2 : Sum  Inputs=|++++
  disturbance2 : Subsystem
  disturbance3 : Subsystem
  old disturbance : Subsystem
  disturbance : Outport
  wires:
  Sum2/1 -> MATLAB Function/1(u)
  Gain1/1 -> Sum2/1
  disturbance2/1(Out1) -> Gain2/1
  a/1 -> disturbance3/1(a)
  a1/1 -> disturbance3/2(a1)
  disturbance3/1(d) -> Gain1/1
  Gain2/1 -> Sum2/2
  old disturbance/1(Out1) -> Gain3/1
  Gain3/1 -> Sum2/3
  MATLAB Function/1(y) -> disturbance/1
  Input/1 -> MATLAB Function/2(d)
  Input1/1 -> MATLAB Function1/1(u)
  MATLAB Function1/1(d) -> Scope/1, Gain4/1
  Gain4/1 -> Sum2/4

== system simulation_Hippocampus_compare_paper/NDI/HippCampus1 ==
  input : Inport
  disturbance : Inport  Port=2
  Controls: Angular Velocities : Scope
  Controls: Rotors1 : Scope
  Controls: Torques : Scope
  Display : Display
  Display1 : Display
  HippoCampus : MATLAB Function  TreatAsAtomicUnit=on
  Integrator : Integrator  InitialCondition=[0; 0; 0; 0;0;0;zeros(6,1)]
  Subsystem : Subsystem
  Subsystem1 : Subsystem
  Subsystem4 : Subsystem
  Sum : Sum  Inputs=|++
  To Workspace8 : ToWorkspace  VariableName=u_NDI  SaveFormat=Timeseries  SampleTime=-1
  sat2 : MATLAB Function  TreatAsAtomicUnit=on
  state : Outport
  wires:
  HippoCampus/1(dx) -> Sum/1  "dx"
  Sum/1 -> Integrator/1
  sat2/2(omega) -> Controls: Angular Velocities/1
  input/1 -> sat2/1(u), Controls: Rotors1/1
  disturbance/1 -> Sum/2
  Integrator/1 -> Subsystem/1(In1)
  Subsystem/1(state) -> state/1, HippoCampus/1(x)
  sat2/1(u_sat) -> To Workspace8/1, Subsystem4/1(u), Subsystem1/1(u), HippoCampus/2(in), Controls: Torques/1
  Subsystem4/1(Out1) -> Display1/1
  Subsystem1/1(Out1) -> Display/1

== system simulation_Hippocampus_compare_paper/NDI4/Controller ==
  r : Inport
  x : Inport  Port=2
  Constant : Constant  Value=k_pos_ndi
  Constant1 : Constant  Value=k_vel_ndi
  Demux1 : Demux  Outputs=[3 3 3 3]
  Gain : Gain  Gain=[ eye(3); zeros(3) ]  Multiplication=Matrix(K*u) (u vector)
  MATLAB Function : MATLAB Function  TreatAsAtomicUnit=on
  Mux1 : Mux  Inputs=2
  Pos controller1 : MATLAB Function  TreatAsAtomicUnit=on
  Saturation : Saturate  UpperLimit=8  LowerLimit=-8
  Scope : Scope
  Subsystem : Subsystem
  Subsystem1 : Subsystem
  Terminator1 : Terminator
  Terminator4 : Terminator
  u : Outport
  wires:
  Subsystem/1(tau) -> u/1
  Constant/1 -> Pos controller1/3(k_pos)
  r/1 -> Gain/1
  Constant1/1 -> Pos controller1/4(k_vel)
  Demux1/3 -> Mux1/2
  Subsystem1/1(x_2pi) -> Demux1/1, MATLAB Function/2(x), Subsystem/3(state)
  Mux1/1 -> Pos controller1/2(x)
  Gain/1 -> Pos controller1/1(r)
  Demux1/1 -> Mux1/1
  Pos controller1/1(u) -> Scope/1, Saturation/1
  Pos controller1/2(theta_des) -> MATLAB Function/1("theta_des ")
  Demux1/2 -> Terminator4/1
  Demux1/4 -> Terminator1/1
  x/1 -> Subsystem1/1(x)
  MATLAB Function/1(theta_des) -> Subsystem/2(rpy_ref)
  Saturation/1 -> Subsystem/1(u_ref)

== system simulation_Hippocampus_compare_paper/NDI4/Disturbance: All derivatives1 ==
  a : Inport
  a1 : Inport  Port=2
  Gain1 : Gain  Gain=0  Multiplication=Matrix(K*u)
  Gain2 : Gain  Multiplication=Matrix(K*u)
  Gain3 : Gain  Gain=0  Multiplication=Matrix(K*u)
  Sum2 : Sum  Inputs=|+++
  disturbance2 : Subsystem
  disturbance3 : Subsystem
  old disturbance : Subsystem
  disturbance : Outport
  wires:
  Sum2/1 -> disturbance/1
  Gain1/1 -> Sum2/1
  disturbance2/1(Out1) -> Gain2/1
  a/1 -> disturbance3/1(a)
  a1/1 -> disturbance3/2(a1)
  disturbance3/1(d) -> Gain1/1
  Gain2/1 -> Sum2/2
  old disturbance/1(Out1) -> Gain3/1
  Gain3/1 -> Sum2/3

== system simulation_Hippocampus_compare_paper/NDI4/Disturbance: All derivatives2 ==
  a : Inport
  a1 : Inport  Port=2
  Input : Inport  Port=3
  Input1 : Inport  Port=4
  Gain1 : Gain  Gain=0  Multiplication=Matrix(K*u)
  Gain2 : Gain  Multiplication=Matrix(K*u)
  Gain3 : Gain  Gain=0  Multiplication=Matrix(K*u)
  Gain4 : Gain  Gain=0  Multiplication=Matrix(K*u)
  MATLAB Function : MATLAB Function  TreatAsAtomicUnit=on
  MATLAB Function1 : MATLAB Function  TreatAsAtomicUnit=on
  Scope : Scope
  Sum2 : Sum  Inputs=|++++
  disturbance2 : Subsystem
  disturbance3 : Subsystem
  old disturbance : Subsystem
  disturbance : Outport
  wires:
  Sum2/1 -> MATLAB Function/1(u)
  Gain1/1 -> Sum2/1
  disturbance2/1(Out1) -> Gain2/1
  a/1 -> disturbance3/1(a)
  a1/1 -> disturbance3/2(a1)
  disturbance3/1(d) -> Gain1/1
  Gain2/1 -> Sum2/2
  old disturbance/1(Out1) -> Gain3/1
  Gain3/1 -> Sum2/3
  MATLAB Function/1(y) -> disturbance/1
  Input/1 -> MATLAB Function/2(d)
  Input1/1 -> MATLAB Function1/1(u)
  MATLAB Function1/1(d) -> Scope/1, Gain4/1
  Gain4/1 -> Sum2/4

== system simulation_Hippocampus_compare_paper/NDI4/HippCampus1 ==
  input : Inport
  disturbance : Inport  Port=2
  Controls: Angular Velocities : Scope
  Controls: Rotors1 : Scope
  Controls: Torques : Scope
  Display : Display
  Display1 : Display
  HippoCampus : MATLAB Function  TreatAsAtomicUnit=on
  Integrator : Integrator  InitialCondition=[0; 0; 0; 0;0;0;zeros(6,1)]
  Subsystem : Subsystem
  Subsystem1 : Subsystem
  Subsystem4 : Subsystem
  Sum : Sum  Inputs=|++
  To Workspace8 : ToWorkspace  VariableName=u_NDI  SaveFormat=Timeseries  SampleTime=-1
  state : Outport
  wires:
  HippoCampus/1(dx) -> Sum/1  "dx"
  Sum/1 -> Integrator/1
  ? -> Controls: Angular Velocities/1
  disturbance/1 -> Sum/2
  Integrator/1 -> Subsystem/1(In1)
  Subsystem/1(state) -> state/1, HippoCampus/1(x)
  input/1 -> To Workspace8/1, Subsystem4/1(u), Subsystem1/1(u), HippoCampus/2(in), Controls: Torques/1, Controls: Rotors1/1
  Subsystem4/1(Out1) -> Display1/1
  Subsystem1/1(Out1) -> Display/1

== system simulation_Hippocampus_compare_paper/PDPD/Controller ==
  r : Inport
  x : Inport  Port=2
  Constant : Constant  Value=8
  Constant1 : Constant  Value=6
  Demux : Demux  Outputs=3
  Demux1 : Demux  Outputs=[3 3 3 3]
  Demux2 : Demux  Outputs=3
  Gain : Gain  Gain=[ eye(3); zeros(3) ]  Multiplication=Matrix(K*u) (u vector)
  Gain1 : Gain  Gain=[ eye(3); zeros(3) ]  Multiplication=Matrix(K*u) (u vector)
  MATLAB Function : MATLAB Function  TreatAsAtomicUnit=on
  Mux1 : Mux  Inputs=2
  Mux2 : Mux  Inputs=2
  Mux4 : Mux  Inputs=2
  PD for linearized attitude dynamics : MATLAB Function  TreatAsAtomicUnit=on
  Pos controller : MATLAB Function  TreatAsAtomicUnit=on
  Scope : Scope
  Scope1 : Scope
  Subsystem1 : Subsystem
  Sum : Sum  Inputs=|+-
  d gains : Constant  Value=[3;8;8]
  p gains : Constant  Value=[20;20;20]
  u : Outport
  wires:
  Mux1/1 -> u/1  "u"
  Pos controller/1(u) -> Mux1/1
  x/1 -> Subsystem1/1(x)
  Demux1/1 -> Mux4/1
  Demux1/3 -> Mux4/2
  Mux4/1 -> Pos controller/2(x)
  Demux1/2 -> Mux2/1
  Demux1/4 -> Mux2/2
  Mux2/1 -> PD for linearized attitude dynamics/2(x)
  Pos controller/2(theta_des) -> MATLAB Function/1("theta_des ")
  Gain1/1 -> PD for linearized attitude dynamics/1(r)
  PD for linearized attitude dynamics/2(u_hs) -> Sum/2, Scope1/1
  PD for linearized attitude dynamics/1(u) -> Sum/1, Scope/1
  Sum/1 -> Mux1/2
  r/1 -> Gain/1
  Gain/1 -> Pos controller/1(r)
  Constant/1 -> Pos controller/3(k_pos)
  Constant1/1 -> Pos controller/4(k_vel)
  p gains/1 -> Demux/1
  Demux/1 -> PD for linearized attitude dynamics/3(p_roll)
  Demux/2 -> PD for linearized attitude dynamics/4(p_pitch)
  Demux/3 -> PD for linearized attitude dynamics/5(p_yaw)
  d gains/1 -> Demux2/1
  Demux2/1 -> PD for linearized attitude dynamics/6(d_roll)
  Demux2/2 -> PD for linearized attitude dynamics/7(d_pitch)
  Demux2/3 -> PD for linearized attitude dynamics/8(d_yaw)
  MATLAB Function/1(theta_des) -> Gain1/1
  Subsystem1/1(x_2pi) -> MATLAB Function/2(x), Demux1/1

== system simulation_Hippocampus_compare_paper/PDPD/Disturbance: All derivatives1 ==
  a : Inport
  a1 : Inport  Port=2
  Input : Inport  Port=3
  Gain1 : Gain  Gain=0  Multiplication=Matrix(K*u)
  Gain2 : Gain  Multiplication=Matrix(K*u)
  Gain3 : Gain  Gain=0  Multiplication=Matrix(K*u)
  MATLAB Function : MATLAB Function  TreatAsAtomicUnit=on
  Sum2 : Sum  Inputs=|+++
  disturbance2 : Subsystem
  disturbance3 : Subsystem
  old disturbance : Subsystem
  disturbance : Outport
  wires:
  Sum2/1 -> MATLAB Function/1(u)
  Gain1/1 -> Sum2/1
  disturbance2/1(Out1) -> Gain2/1
  a/1 -> disturbance3/1(a)
  a1/1 -> disturbance3/2(a1)
  disturbance3/1(d) -> Gain1/1
  Gain2/1 -> Sum2/2
  old disturbance/1(Out1) -> Gain3/1
  Gain3/1 -> Sum2/3
  MATLAB Function/1(y) -> disturbance/1
  Input/1 -> MATLAB Function/2(d)

== system simulation_Hippocampus_compare_paper/PDPD/HippCampus1 ==
  input : Inport
  disturbance : Inport  Port=2
  Controls: Angular Velocities : Scope
  Controls: Rotors1 : Scope
  Controls: Torques : Scope
  Display : Display
  Display1 : Display
  HippoCampus : MATLAB Function  TreatAsAtomicUnit=on
  Integrator : Integrator  InitialCondition=[0; 0; 0; 0;0;0;zeros(6,1)]
  Subsystem : Subsystem
  Subsystem1 : Subsystem
  Subsystem4 : Subsystem
  Sum : Sum  Inputs=|++
  To Workspace8 : ToWorkspace  VariableName=u_PDPD  SaveFormat=Timeseries  SampleTime=-1
  sat1 : MATLAB Function  TreatAsAtomicUnit=on
  state : Outport
  wires:
  HippoCampus/1(dx) -> Sum/1  "dx"
  Sum/1 -> Integrator/1
  ? -> Controls: Angular Velocities/1
  disturbance/1 -> Sum/2
  Integrator/1 -> Subsystem/1(In1)
  Subsystem/1(state) -> state/1, HippoCampus/1(x)
  Subsystem4/1(Out1) -> Display1/1
  Subsystem1/1(Out1) -> Display/1
  sat1/1(u_sat) -> Subsystem4/1(u), To Workspace8/1, Subsystem1/1(u), HippoCampus/2(in), Controls: Torques/1, Controls: Rotors1/1
  input/1 -> sat1/1(u)

== system simulation_Hippocampus_compare_paper/PDPD1/Controller ==
  r : Inport
  x : Inport  Port=2
  Constant : Constant  Value=8
  Constant1 : Constant  Value=8
  Demux : Demux  Outputs=3
  Demux1 : Demux  Outputs=[3 3 3 3]
  Demux2 : Demux  Outputs=3
  Gain : Gain  Gain=[ eye(3); zeros(3) ]  Multiplication=Matrix(K*u) (u vector)
  Gain1 : Gain  Gain=[ eye(3); zeros(3) ]  Multiplication=Matrix(K*u) (u vector)
  MATLAB Function : MATLAB Function  TreatAsAtomicUnit=on
  Mux1 : Mux  Inputs=2
  Mux2 : Mux  Inputs=2
  Mux4 : Mux  Inputs=2
  PD for linearized attitude dynamics : MATLAB Function  TreatAsAtomicUnit=on
  Pos controller : MATLAB Function  TreatAsAtomicUnit=on
  Scope : Scope
  Scope1 : Scope
  Subsystem1 : Subsystem
  Sum : Sum  Inputs=|+-
  d gains : Constant  Value=[3;8;8]
  p gains : Constant  Value=[20;20;20]
  u : Outport
  wires:
  Mux1/1 -> u/1  "u"
  Pos controller/1(u) -> Mux1/1
  x/1 -> Subsystem1/1(x)
  Demux1/1 -> Mux4/1
  Demux1/3 -> Mux4/2
  Mux4/1 -> Pos controller/2(x)
  Demux1/2 -> Mux2/1
  Demux1/4 -> Mux2/2
  Mux2/1 -> PD for linearized attitude dynamics/2(x)
  Pos controller/2(theta_des) -> MATLAB Function/1("theta_des ")
  Gain1/1 -> PD for linearized attitude dynamics/1(r)
  PD for linearized attitude dynamics/2(u_hs) -> Sum/2, Scope1/1
  PD for linearized attitude dynamics/1(u) -> Sum/1, Scope/1
  Sum/1 -> Mux1/2
  r/1 -> Gain/1
  Gain/1 -> Pos controller/1(r)
  Constant/1 -> Pos controller/3(k_pos)
  Constant1/1 -> Pos controller/4(k_vel)
  p gains/1 -> Demux/1
  Demux/1 -> PD for linearized attitude dynamics/3(p_roll)
  Demux/2 -> PD for linearized attitude dynamics/4(p_pitch)
  Demux/3 -> PD for linearized attitude dynamics/5(p_yaw)
  d gains/1 -> Demux2/1
  Demux2/1 -> PD for linearized attitude dynamics/6(d_roll)
  Demux2/2 -> PD for linearized attitude dynamics/7(d_pitch)
  Demux2/3 -> PD for linearized attitude dynamics/8(d_yaw)
  MATLAB Function/1(theta_des) -> Gain1/1
  Subsystem1/1(x_2pi) -> MATLAB Function/2(x), Demux1/1

== system simulation_Hippocampus_compare_paper/PDPD1/Disturbance: All derivatives1 ==
  a : Inport
  a1 : Inport  Port=2
  Input : Inport  Port=3
  Gain1 : Gain  Gain=0  Multiplication=Matrix(K*u)
  Gain2 : Gain  Multiplication=Matrix(K*u)
  Gain3 : Gain  Gain=0  Multiplication=Matrix(K*u)
  MATLAB Function : MATLAB Function  TreatAsAtomicUnit=on
  Sum2 : Sum  Inputs=|+++
  disturbance2 : Subsystem
  disturbance3 : Subsystem
  old disturbance : Subsystem
  disturbance : Outport
  wires:
  Sum2/1 -> MATLAB Function/1(u)
  Gain1/1 -> Sum2/1
  disturbance2/1(Out1) -> Gain2/1
  a/1 -> disturbance3/1(a)
  a1/1 -> disturbance3/2(a1)
  disturbance3/1(d) -> Gain1/1
  Gain2/1 -> Sum2/2
  old disturbance/1(Out1) -> Gain3/1
  Gain3/1 -> Sum2/3
  MATLAB Function/1(y) -> disturbance/1
  Input/1 -> MATLAB Function/2(d)

== system simulation_Hippocampus_compare_paper/PDPD1/HippCampus1 ==
  input : Inport
  disturbance : Inport  Port=2
  Controls: Angular Velocities : Scope
  Controls: Rotors1 : Scope
  Controls: Torques : Scope
  Display : Display
  Display1 : Display
  HippoCampus : MATLAB Function  TreatAsAtomicUnit=on
  Integrator : Integrator  InitialCondition=[0; 0; 0; 0;0;0;zeros(6,1)]
  Subsystem : Subsystem
  Subsystem1 : Subsystem
  Subsystem4 : Subsystem
  Sum : Sum  Inputs=|++
  To Workspace8 : ToWorkspace  VariableName=u_PDPD  SaveFormat=Timeseries  SampleTime=-1
  state : Outport
  wires:
  HippoCampus/1(dx) -> Sum/1  "dx"
  Sum/1 -> Integrator/1
  ? -> Controls: Angular Velocities/1
  disturbance/1 -> Sum/2
  Integrator/1 -> Subsystem/1(In1)
  Subsystem/1(state) -> state/1, HippoCampus/1(x)
  Subsystem4/1(Out1) -> Display1/1
  Subsystem1/1(Out1) -> Display/1
  input/1 -> Subsystem4/1(u), To Workspace8/1, Subsystem1/1(u), HippoCampus/2(in), Controls: Torques/1, Controls: Rotors1/1
